simulink model "BalancingModel_24a"  (R2024a)
settings: Solver=FixedStepDiscrete  StartTime=0.0  StopTime=inf  FixedStep=0.001  RelTol=1e-3
settings Model: Creator=Ganna Ayman  LastModifiedBy=Ganna Ayman
settings OptimizationCC: DefaultParameterBehavior=Inlined  UseDivisionForNetSlopeComputation=on  GainParamInheritBuiltInType=on  UseFloatMulNetSlope=on  InlineInvariantSignals=on  PassReuseOutputArgsAs=Individual arguments  ZeroExternalMemoryAtStartup=off  ZeroInternalMemoryAtStartup=off  NoFixptDivByZeroProtection=on  EfficientFloat2IntCast=on  LifeSpan=1  OptimizeBlockOrder=speed  DifferentSizesBufferReuse=on  EfficientTunableParamExpr=on
settings DebuggingCC: ParameterTunabilityLossMsg=error
settings HardwareCC: ProdBitPerPointer=32  ProdBitPerSizeT=32  ProdBitPerPtrDiffT=32  ProdLargestAtomicInteger=Long  ProdLargestAtomicFloat=Double  ProdWordSize=32  ProdLongLongMode=on  ProdHWDeviceType=NXP->Cortex-M0/M0+
settings SFSimCC: MATLABDynamicMemAlloc=off
settings RTWCC: Description=Embedded Coder  SystemTargetFile=ert.tlc  TemplateMakefile=ert_default_tmf
settings CodeAppCC: ForceParamTrailComments=on  IgnoreCustomStorageClasses=off  OperatorAnnotations=on  SimulinkDataObjDesc=on  SFDataObjDesc=on  CustomSymbolStrGlobalVar=rt$N$M  CustomSymbolStrType=$N$M  CustomSymbolStrFcn=$N$M$F  CustomSymbolStrMacro=$N$M  InsertBlockDesc=on
settings ERTTargetCC: TargetLangStandard=C99 (ISO)  GenerateSampleERTMain=on  IncludeMdlTerminateFcn=off  CombineSignalStateStructs=on  SupportAbsoluteTime=off  SupportComplex=off  SupportNonInlinedSFcns=on  InlinedParameterPlacement=NonHierarchical  ERTCustomFileTemplate=example_file_process.tlc  ERTFilePackagingFormat=CompactWithDataFile

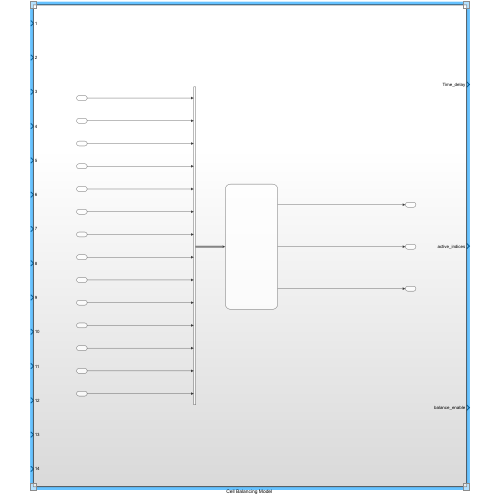
[thumbnail: Simulink's stored preview of the top-level diagram]
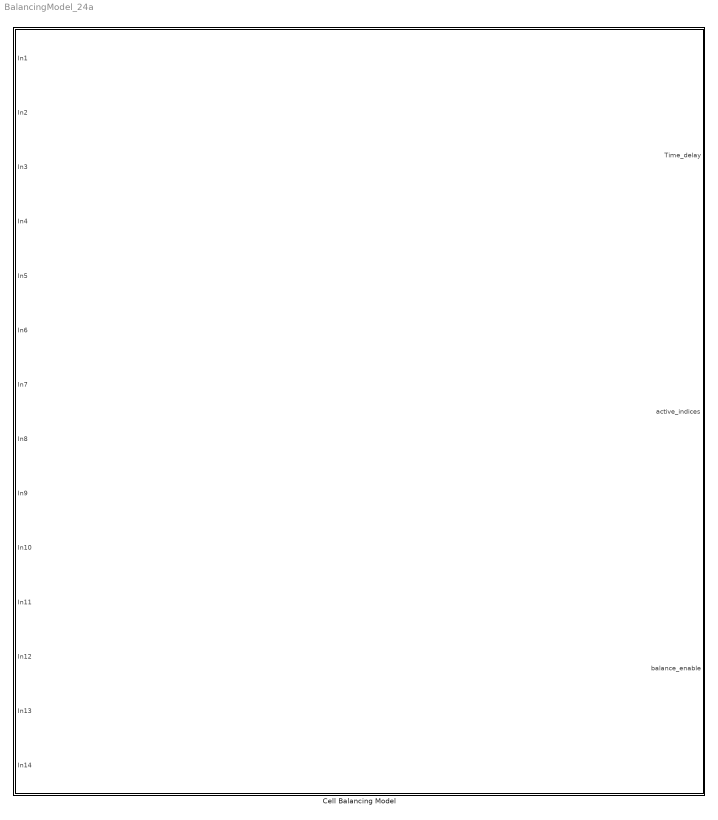
== system BalancingModel_24a ==
  "Cell Balancing Model " : Subsystem

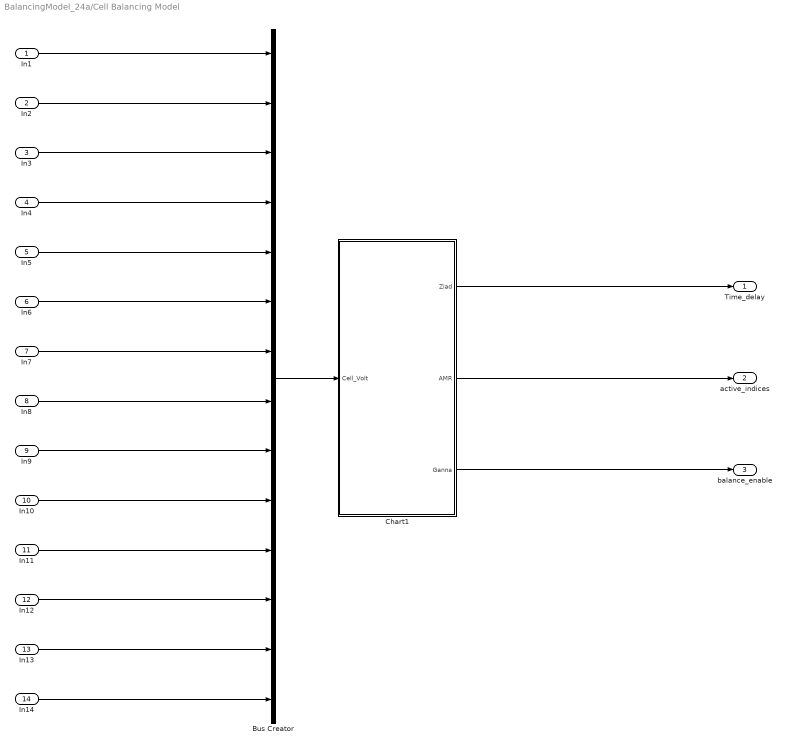
== system BalancingModel_24a/Cell Balancing Model  ==
  In1 : Inport
  In2 : Inport  Port=2
  In3 : Inport  Port=3
  In4 : Inport  Port=4
  In5 : Inport  Port=5
  In6 : Inport  Port=6
  In7 : Inport  Port=7
  In8 : Inport  Port=8
  In9 : Inport  Port=9
  In10 : Inport  Port=10
  In11 : Inport  Port=11
  In12 : Inport  Port=12
  In13 : Inport  Port=13
  In14 : Inport  Port=14
  Bus Creator : BusCreator  Inputs=14
  Chart1 : Stateflow chart  TreatAsAtomicUnit=on
      settings: PortSchema="{\"entries\":[{\"content\":{\"sides\":[{\"content\":{\"connectorIds\":[\"In1\"]},\"type\":\"ConnectorPlacement.EquallySpacedRectSide\",\"uuid\":\"6f312cc7-79af-4024-8579-3732173f9295\"},{\"content\":{\"connectorIds\":[\"Out2\",\"Out3\",\"Out1\"],\"side\":\"RIGHT\"},\"type\":\"ConnectorPlacement.EquallySpacedRectSide\",\"uuid\":\"3dc9c74e-fd1a-461c-96fc-bb153941e7b5\"},{\"content\":{\"side\":\"TOP\"},\"type\":\"ConnectorPlacement.EquallySpacedRectSide\",\"uuid\":\"e4504d25-18f4-45f4-b711-d682a6c51dcf\"}]},\"type\":\"ConnectorPlacement.EquallySpacedConnector\",\"uuid\":\"9caf59e1-89f7-43be-b634-7a97cd583662\"}],\"packageUris\":[\"http://schema.mathworks.com/mf0/Connector/R2020b\"],\"version\":\"1.0\"}"
  Time_delay : Outport
  active_indices : Outport  Port=2
  balance_enable : Outport  Port=3
  wires:
  In10/1 -> Bus Creator/10
  In5/1 -> Bus Creator/5
  In13/1 -> Bus Creator/13
  In7/1 -> Bus Creator/7
  In14/1 -> Bus Creator/14
  In1/1 -> Bus Creator/1
  In9/1 -> Bus Creator/9
  In2/1 -> Bus Creator/2
  In3/1 -> Bus Creator/3
  Chart1/2(Ziad) -> Time_delay/1
  Chart1/3(AMR) -> active_indices/1
  In11/1 -> Bus Creator/11
  In8/1 -> Bus Creator/8
  In4/1 -> Bus Creator/4
  In12/1 -> Bus Creator/12
  In6/1 -> Bus Creator/6
  Chart1/1(Ganna) -> balance_enable/1
  Bus Creator/1 -> Chart1/1(Cell_Volt)

== stateflow chart BalancingModel_24a/Cell Balancing Model /Chart1 ==
  state Discharge_Time_interval
    H= 1;
    Ziad = zeros(1, 14);  % Initialize array
    during:
    for H = 1:14
    if    Ganna(H) == 1
    Ziad(H) = 0.5; % 0.5min
    else
    Ziad(H) = 0;      % 0 if disabled
    end
    end
    exit:
    H=1;
  state initialization
    entry:
    Ganna=zeros(1,14);
    n=1;
    i=1;
    G=1;
    H=1;
  state Get_balance_reference
    entry:
    i=1
    cell_reference=10;
    during :
    for i = 1:14
    if (Cell_Volt(i) < cell_reference) && (Cell_Volt(i)>1.5)
    cell_reference = Cell_Volt(i);
    end
    end;
    exit:
    i=1;
  state Index_number
    entry:
    AMR = zeros(1,14);  % Initialize output
    idx = 1;                     % Counter for active indices
    during:
    for G = 1:14
    if    Ganna(G) == 1
    AMR(idx) = G;  % Store cell
    idx = idx + 1;
    end
    end
    exit:
    G=1;
  state Data_Check
    i = 1;
    % Main loop
    for i = 1:14
    if (Cell_Volt(i) > cell_reference) && (Cell_Volt(i) > 1.6) &&(Cell_Volt(i) - cell_reference > 0.25)
    Ganna(i) = 1;
    else
    Ganna(i) = 0; %had5ol feha 3and as8ar wa7da + lo el difference kan akber mn 0.25
    end
    end
    exit :
    i=1;
  state Error_Check
    entry:
    abdullah = 0;  % Initialize output (0 by default)
    during:
    for G = 1:14
    % Calculate absolute difference
    diff = abs(Cell_Volt(G) - cell_reference);
    % Check condition
    if diff > 0.5
    abdullah = 1;  % Set flag
    end
    end
    end
    exit:
    G=1;
  (default) -> initialization
  Discharge_Time_interval -> Get_balance_reference : after(30,sec)[(H==14)]
  initialization -> Get_balance_reference
  Index_number -> Discharge_Time_interval : [G==14]
  Error_Check -> Get_balance_reference [order 2] : [abdullah==1]
  Get_balance_reference -> Error_Check : [i==14]
  Data_Check -> Index_number : [i==14]
  Error_Check -> Data_Check [order 1] : [(G==14)&&(abdullah==0)]
  data: Cell_Volt input double size=[1,14]; Ganna output double size=[1,14]; i local; G local; H local; n local; cell_reference local; Ziad output double size=[1,14]; AMR output double size=[1,14]; idx local; abdullah local; diff local
